simulink model "m_2b_simulink"  (R2021b)
settings: Solver=VariableStepAuto  StartTime=0.0  StopTime=10  RelTol=1e-6
values from neighbouring files (symbols this model uses):
  g = 9.81    [m_2b_matlab.m]
  l = 4    [m_2b_matlab.m]
  m = 1    [m_2b_matlab.m]
settings Model: Creator=Brad  LastModifiedBy=Brad

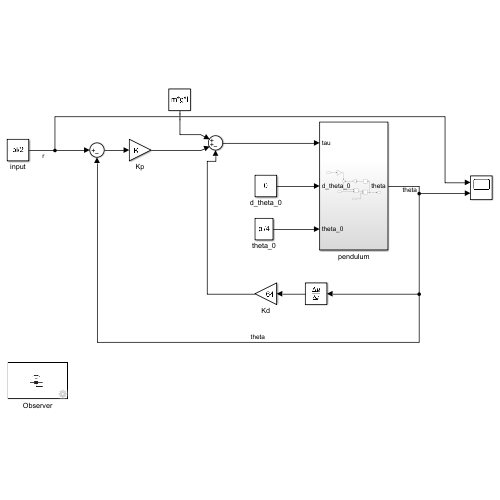
[thumbnail: Simulink's stored preview of the top-level diagram]
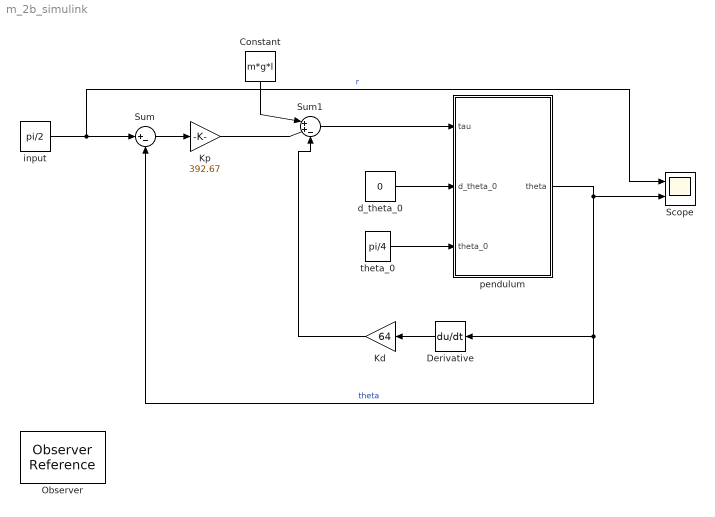
== system m_2b_simulink ==
  Constant : Constant  Value=m*g*l
  Derivative : Derivative
  Kd : Gain  Gain=64
  Kp : Gain  Gain=392.67
  Observer : ObserverReference  ObserverModelName=m_2b_simulink_Observer1
  Scope : Scope  NumInputPorts=2
  Sum : Sum  Inputs=|+-
  Sum1 : Sum  Inputs=|++-
  d_theta_0 : Constant  Value=0
  input : Constant  Value=pi/2
  pendulum : Subsystem
  theta_0 : Constant  Value=pi/4  VectorParams1D=off
  wires:
  d_theta_0/1 -> pendulum/2(d_theta_0)
  input/1 -> Scope/1, Sum/1  "r"
  pendulum/1(theta) -> Derivative/1, Sum/2, Scope/2  "theta"
  Kp/1 -> Sum1/2
  Sum/1 -> Kp/1
  Sum1/1 -> pendulum/1(tau)
  Kd/1 -> Sum1/3
  Derivative/1 -> Kd/1
  theta_0/1 -> pendulum/3(theta_0)
  Constant/1 -> Sum1/1

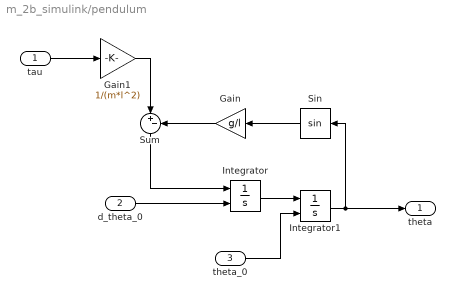
== system m_2b_simulink/pendulum ==
  tau : Inport
  d_theta_0 : Inport  Port=2
  theta_0 : Inport  Port=3
  Gain : Gain  Gain=g/l
  Gain1 : Gain  Gain=1/(m*l^2)
  Integrator : Integrator  InitialConditionSource=external
  Integrator1 : Integrator  InitialConditionSource=external  InitialCondition=pi/4
  Sin : Trigonometry
  Sum : Sum  Inputs=|+-
  theta : Outport
  wires:
  Sin/1 -> Gain/1
  Gain/1 -> Sum/2
  Sum/1 -> Integrator/1
  Integrator1/1 -> Sin/1, theta/1
  Integrator/1 -> Integrator1/1
  tau/1 -> Gain1/1
  Gain1/1 -> Sum/1
  d_theta_0/1 -> Integrator/2
  theta_0/1 -> Integrator1/2
